simulink model "and_state_interleavings_2_1"  (Simulink 6.6)
settings: Solver=FixedStepDiscrete  StartTime=0.0  StopTime=10.0  FixedStep=1  RelTol=1e-3
settings Model: Creator=vBuskirk  LastModifiedBy=vBuskirk

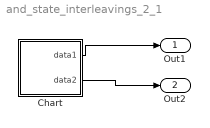
== system and_state_interleavings_2_1 ==
  Chart : Stateflow chart
  Out1 : Outport
  Out2 : Outport  Port=2
  wires:
  Chart/1(data1) -> Out1/1
  Chart/2(data2) -> Out2/1

== stateflow chart Chart ==
  state Parent1 [parallel]
    settings: executionOrder=2
    state S3 [parallel]
      settings: executionOrder=3
      state S3_a
      state S3_c
        en: data1=4;
      state S3_b
        en: data1=3;
      (default) -> Parent1.S3.S3_a
      Parent1.S3.S3_a -> Parent1.S3.S3_b [order 2] : [data1==1]
      Parent1.S3.S3_a -> Parent1.S3.S3_c [order 1] : [data1==2]
    state S2 [parallel]
      en: data1 = 2;
      settings: executionOrder=1
    state S1 [parallel]
      en: data1 = 1;
      settings: executionOrder=2
  state Parent2 [parallel]
    settings: executionOrder=1
    state S2 [parallel]
      en: data2 = 2;
      settings: executionOrder=1
    state S1 [parallel]
      en: data2 = 1;
      settings: executionOrder=2
    state S3 [parallel]
      settings: executionOrder=3
      state S3_a
      state S3_c
        en: data2=4;
      state S3_b
        en: data2=3;
      (default) -> Parent2.S3.S3_a
      Parent2.S3.S3_a -> Parent2.S3.S3_b [order 2] : [data2==1]
      Parent2.S3.S3_a -> Parent2.S3.S3_c [order 1] : [data2==2]
  data: data1 output double; data2 output double
